simulink model "gm_rgbFilter_2024a"  (R2024a)
settings: Solver=FixedStepDiscrete  StartTime=0.0  StopTime=2  RelTol=1e-3
undefined symbols (not defined in the file or in its folder): blueMax, gray, greenMax, redMax
libraries: hdlsllib x13, visionhdlio x3, visionsources x1
Description:
  | Sobel Edge Detection Using the MATLAB(R) Function Block
  | This example shows how to use HDL Coder(TM) to check,
  | generate, and verify HDL code for a Sobel Edge Detection
  | block built using the MATLAB Function block.
settings Model: FPTRunName=Active  Creator=The MathWorks, Inc.  LastModifiedBy=dskiee
settings SolverCC: AlgebraicLoopSolver=TrustRegion
settings DataIOCC: LimitDataPoints=on  SaveFormat=Array  SignalLogging=off  ReturnWorkspaceOutputs=off
settings OptimizationCC: BlockReduction=off  ConditionallyExecuteInputs=off  DefaultParameterBehavior=Inlined  ExpressionDepthLimit=2147483647  InitFltsAndDblsToZero=on  EfficientMapNaN2IntZero=off  LifeSpan=inf
settings DebuggingCC: AlgebraicLoopMsg=error  SaveWithParameterizedLinksMsg=none  UnderspecifiedInitializationDetection=Classic  MergeDetectMultiDrivingBlocksExec=none  SignalResolutionControl=TryResolveAllWithWarning  InheritedTsInSrcMsg=none  MultiTaskDSMMsg=warning  MultiTaskCondExecSysMsg=none  SingleTaskRateTransMsg=error  IntegerOverflowMsg=none  ParameterPrecisionLossMsg=none  FcnCallInpInsideContextMsg=warning  UnconnectedInputMsg=warning  UnconnectedOutputMsg=warning  UnconnectedLineMsg=warning  AllowSymbolicDim=off  StateNameClashWarn=warning  StrictBusMsg=ErrorOnBusTreatedAsVector  SFUnexpectedBacktrackingDiag=warning  SFNoUnconditionalDefaultTransitionDiag=warning  SFExecutionAtInitializationDiag=none  IntegerSaturationMsg=none  ArithmeticOperatorsInVariantConditions=warning
settings HardwareCC: ProdBitPerPointer=32  ProdBitPerSizeT=32  ProdBitPerPtrDiffT=32  ProdLargestAtomicFloat=None  ProdIntDivRoundTo=Undefined  ProdEndianess=Unspecified  ProdWordSize=32  ProdHWDeviceType=ASIC/FPGA  TargetHWDeviceType=32-bit Generic  ProdEqTarget=off
settings ModelReferenceCC: EnableRefExpFcnMdlSchedulingChecks=on  PropagateSignalLabelsOutOfModel=off
settings SFSimCC: SimUseLocalCustomCode=off  CustomCodeUndefinedFunction=UseInterfaceOnly
settings RTWCC: RTWUseLocalCustomCode=off  GPUComputeCapability=3.5  DLArmComputeVersion=19.05
settings CodeAppCC: StateflowObjectComments=on
settings GRTTargetCC: TargetFcnLib=ansi_tfl_tmw.mat  TargetLangStandard=C89/C90 (ANSI)  CombineOutputUpdateFcns=off  GRTInterface=on
settings ConfigComp: CovMetricSettings=dw  CovSaveCumulativeToWorkspaceVar=on  CovSaveSingleToWorkspaceVar=on  CovExternalEMLEnable=off

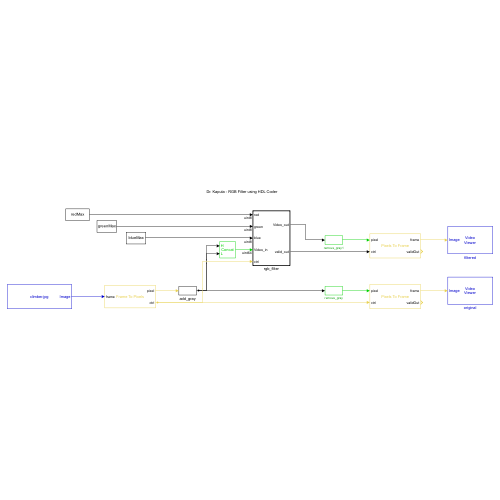
[thumbnail: Simulink's stored preview of the top-level diagram]
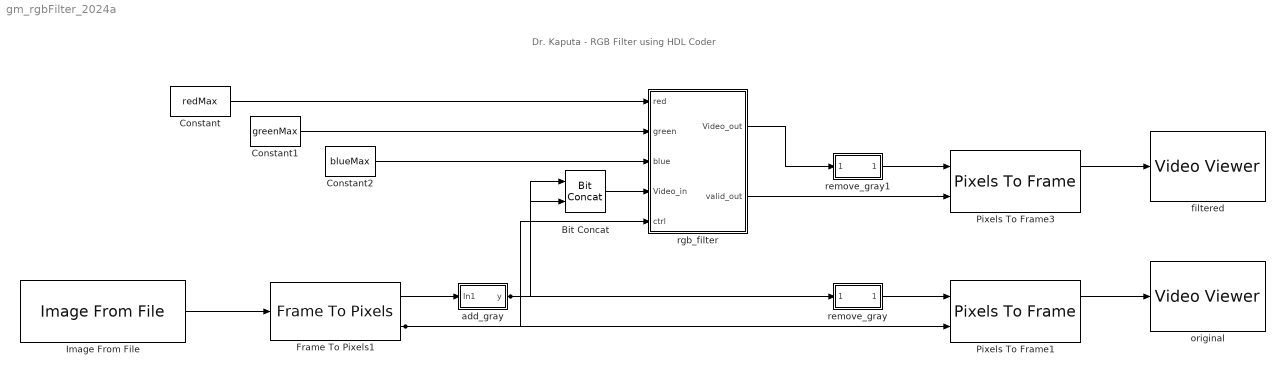
== system gm_rgbFilter_2024a ==
  note: Dr. Kaputa - RGB Filter using HDL Coder
  Bit Concat : hdlsllib/Logic and Bit Operations/Bit Concat  numInputs=2
  Constant : Constant  Value=redMax  OutDataTypeStr=uint8  SampleTime=-1
  Constant1 : Constant  Value=greenMax  OutDataTypeStr=uint8  SampleTime=-1
  Constant2 : Constant  Value=blueMax  OutDataTypeStr=uint8  SampleTime=-1
  Frame To Pixels1 : visionhdlio/Frame To Pixels  NumComponents=3  NumPixels=1  VideoFormat=Custom  ActivePixelsPerLine=R  ActiveVideoLines=C  TotalPixelsPerLine=R  TotalVideoLines=C  StartingActiveLine=1  FrontPorch=0  SampleTime=0  VideoFormatCache=Custom  ActivePixelsPerLineCache=R  ActiveVideoLinesCache=C  TotalPixelsPerLineCache=R  TotalVideoLinesCache=C  StartingActiveLineCache=1  FrontPorchCache=0
  Image From File : visionsources/Image From File  Tag=vipblks_nd  FileName=climber.jpg  Ts=1  imagePorts=One multidimensional signal  OutPortLabels=R|G|B  ImageDataType=Inherit from input image  sdImageDataType=uint(8)  Signed=on  WordLength=16  FractionLengthMode=User-defined  FractionLength=15
  Pixels To Frame1 : visionhdlio/Pixels To Frame  NumComponents=3  NumPixels=1  VideoFormat=Custom  ActivePixelsPerLine=R  ActiveVideoLines=C  TotalPixelsPerLine=R  TotalVideoLines=C  VideoFormatCache=Custom  ActivePixelsPerLineCache=R  ActiveVideoLinesCache=C  TotalPixelsPerLineCache=R  TotalVideoLinesCache=C
  Pixels To Frame3 : visionhdlio/Pixels To Frame  NumComponents=3  NumPixels=1  VideoFormat=Custom  ActivePixelsPerLine=R  ActiveVideoLines=C  TotalPixelsPerLine=R  TotalVideoLines=C  VideoFormatCache=Custom  ActivePixelsPerLineCache=R  ActiveVideoLinesCache=C  TotalPixelsPerLineCache=R  TotalVideoLinesCache=C
  add_gray : Subsystem
  filtered : VideoViewer  colormapValue=gray(256)  FigPos=[-1034.33333333333 813.333333333333 1280 622.666666666667]
  original : VideoViewer  FigPos=[-1388.33333333333 754 1280 622.666666666667]
  remove_gray : Subsystem
  remove_gray1 : Subsystem
  rgb_filter : Subsystem  TreatAsAtomicUnit=on
  wires:
  Constant2/1 -> rgb_filter/3(blue)
  Constant1/1 -> rgb_filter/2(green)
  Constant/1 -> rgb_filter/1(red)
  remove_gray1/1(RGBVector) -> Pixels To Frame3/1
  Bit Concat/1 -> rgb_filter/4(Video_in)
  rgb_filter/2(valid_out) -> Pixels To Frame3/2
  rgb_filter/1(Video_out) -> remove_gray1/1(RGB)
  Pixels To Frame3/1 -> filtered/1
  add_gray/1(y) -> remove_gray/1(RGB), Bit Concat/2, Bit Concat/1
  Frame To Pixels1/1 -> add_gray/1(In1)
  remove_gray/1(RGBVector) -> Pixels To Frame1/1
  Frame To Pixels1/2 -> Pixels To Frame1/2, rgb_filter/5(ctrl)
  Pixels To Frame1/1 -> original/1
  Image From File/1 -> Frame To Pixels1/1

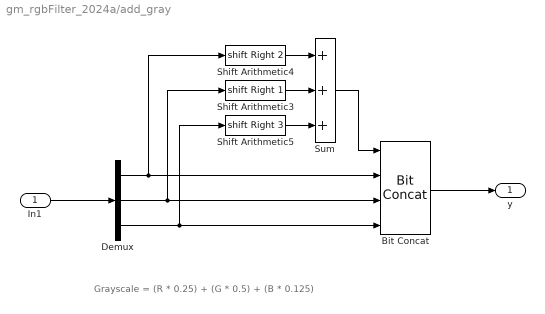
== system gm_rgbFilter_2024a/add_gray ==
  note: Grayscale = (R * 0.25) + (G * 0.5) + (B * 0.125)
  In1 : Inport
  Bit Concat : hdlsllib/Logic and Bit Operations/Bit Concat  numInputs=4
  Demux : Demux  Outputs=3
  Shift Arithmetic3 : ArithShift  BitShiftNumber=1  BitShiftDirection=Right
  Shift Arithmetic4 : ArithShift  BitShiftNumber=2  BitShiftDirection=Right
  Shift Arithmetic5 : ArithShift  BitShiftNumber=3  BitShiftDirection=Right
  Sum : Sum  Inputs=+++  OutDataTypeStr=uint8
  y : Outport
  wires:
  Shift Arithmetic5/1 -> Sum/3
  Shift Arithmetic3/1 -> Sum/2
  Shift Arithmetic4/1 -> Sum/1
  Sum/1 -> Bit Concat/1
  Demux/3 -> Bit Concat/4, Shift Arithmetic5/1
  Demux/1 -> Bit Concat/2, Shift Arithmetic4/1
  Demux/2 -> Bit Concat/3, Shift Arithmetic3/1
  In1/1 -> Demux/1
  Bit Concat/1 -> y/1

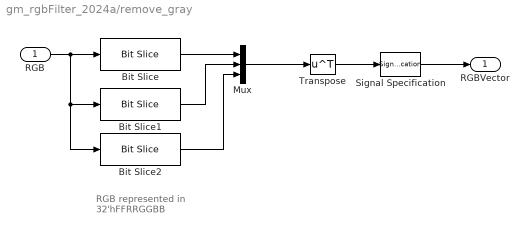
== system gm_rgbFilter_2024a/remove_gray ==
  note: RGB represented in
      | 32'hFFRRGGBB
  RGB : Inport
  Bit Slice : hdlsllib/Logic and Bit Operations/Bit Slice  lidx=23  ridx=16
  Bit Slice1 : hdlsllib/Logic and Bit Operations/Bit Slice  lidx=15  ridx=8
  Bit Slice2 : hdlsllib/Logic and Bit Operations/Bit Slice  lidx=7  ridx=0
  Mux : Mux  Inputs=3
  Signal Specification : SignalSpecification
  Transpose : Math  Operator=transpose  SignedPower=on
  RGBVector : Outport  VectorParamsAs1DForOutWhenUnconnected=off
  wires:
  Mux/1 -> Transpose/1
  Bit Slice/1 -> Mux/1
  Bit Slice2/1 -> Mux/3
  Bit Slice1/1 -> Mux/2
  RGB/1 -> Bit Slice2/1, Bit Slice1/1, Bit Slice/1
  Transpose/1 -> Signal Specification/1
  Signal Specification/1 -> RGBVector/1

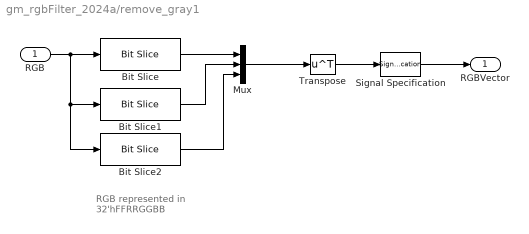
== system gm_rgbFilter_2024a/remove_gray1 ==
  note: RGB represented in
      | 32'hFFRRGGBB
  RGB : Inport
  Bit Slice : hdlsllib/Logic and Bit Operations/Bit Slice  lidx=23  ridx=16
  Bit Slice1 : hdlsllib/Logic and Bit Operations/Bit Slice  lidx=15  ridx=8
  Bit Slice2 : hdlsllib/Logic and Bit Operations/Bit Slice  lidx=7  ridx=0
  Mux : Mux  Inputs=3
  Signal Specification : SignalSpecification
  Transpose : Math  Operator=transpose  SignedPower=on
  RGBVector : Outport  VectorParamsAs1DForOutWhenUnconnected=off
  wires:
  Mux/1 -> Transpose/1
  Bit Slice/1 -> Mux/1
  Bit Slice2/1 -> Mux/3
  Bit Slice1/1 -> Mux/2
  RGB/1 -> Bit Slice2/1, Bit Slice1/1, Bit Slice/1
  Transpose/1 -> Signal Specification/1
  Signal Specification/1 -> RGBVector/1

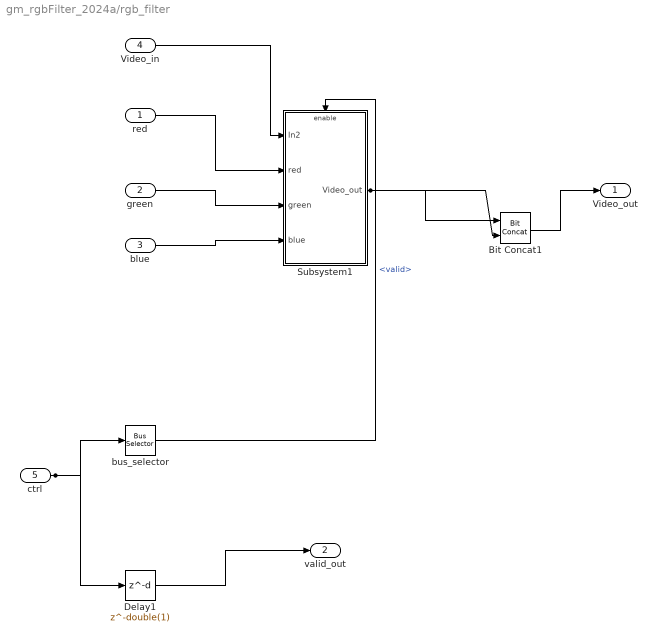
== system gm_rgbFilter_2024a/rgb_filter ==
  red : Inport  OutDataTypeStr=uint8  PortDimensions=1  SampleTime=2.77039007092199e-06
  green : Inport  Port=2  OutDataTypeStr=uint8  PortDimensions=1  SampleTime=2.77039007092199e-06
  blue : Inport  Port=3  OutDataTypeStr=uint8  PortDimensions=1  SampleTime=2.77039007092199e-06
  Video_in : Inport  Port=4  OutDataTypeStr=fixdt(0, 64, 0)  PortDimensions=1  SampleTime=2.77039007092199e-06
  ctrl : Inport  Port=5
  Bit Concat1 : hdlsllib/Logic and Bit Operations/Bit Concat  numInputs=2
  Delay1 : Delay  DelayLength=double(1)  SampleTime=2.77039007092199e-06
  Subsystem1 : Subsystem
  bus_selector : BusSelector  OutputSignals=valid
  Video_out : Outport  SampleTime=2.77039007092199e-06  VectorParamsAs1DForOutWhenUnconnected=off
  valid_out : Outport  Port=2  VectorParamsAs1DForOutWhenUnconnected=off
  wires:
  red/1 -> Subsystem1/2(red)
  green/1 -> Subsystem1/3(green)
  blue/1 -> Subsystem1/4(blue)
  Video_in/1 -> Subsystem1/1(In2)
  ctrl/1 -> bus_selector/1, Delay1/1
  Bit Concat1/1 -> Video_out/1
  bus_selector/1 -> Subsystem1/Enable  "<valid>"
  Delay1/1 -> valid_out/1
  Subsystem1/1(Video_out) -> Bit Concat1/2, Bit Concat1/1

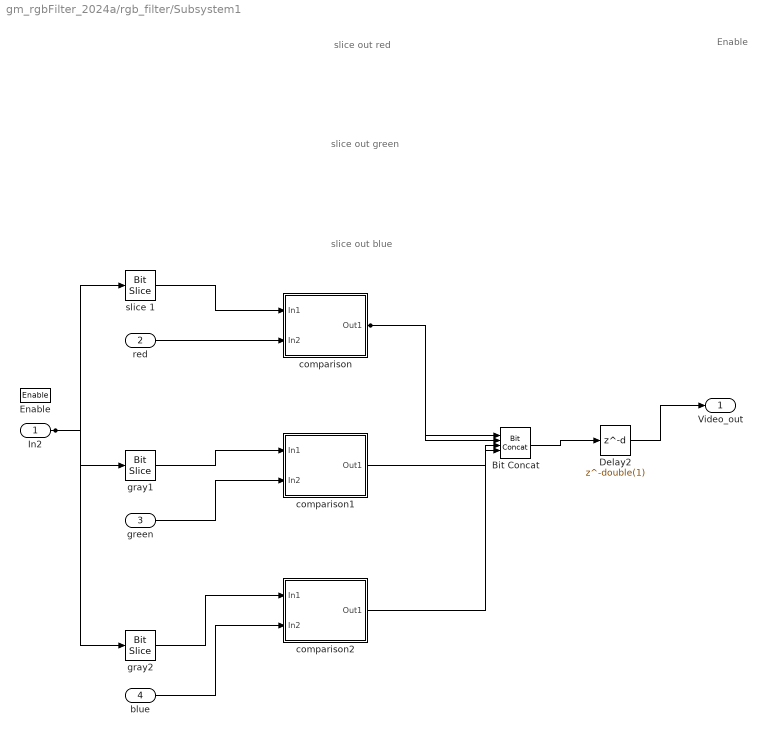
== system gm_rgbFilter_2024a/rgb_filter/Subsystem1 ==
  note: Enable
  note: slice out blue
  note: slice out green
  note: slice out red
  In2 : Inport  OutDataTypeStr=fixdt(0, 64, 0)  PortDimensions=1  SampleTime=2.77039007092199e-06
  red : Inport  Port=2  OutDataTypeStr=uint8  PortDimensions=1  SampleTime=2.77039007092199e-06
  green : Inport  Port=3  OutDataTypeStr=uint8  PortDimensions=1  SampleTime=2.77039007092199e-06
  blue : Inport  Port=4  OutDataTypeStr=uint8  PortDimensions=1  SampleTime=2.77039007092199e-06
  Enable : EnablePort  OutDataTypeStr=boolean
  Bit Concat : hdlsllib/Logic and Bit Operations/Bit Concat  numInputs=4
  Delay2 : Delay  DelayLength=double(1)  InitialCondition=0
  comparison : Subsystem
  comparison1 : Subsystem
  comparison2 : Subsystem
  gray1 : hdlsllib/Logic and Bit Operations/Bit Slice  lidx=double(15)  ridx=double(8)
  gray2 : hdlsllib/Logic and Bit Operations/Bit Slice  lidx=double(7)  ridx=double(0)
  slice 1 : hdlsllib/Logic and Bit Operations/Bit Slice  lidx=double(23)  ridx=double(16)
  Video_out : Outport  SampleTime=2.77039007092199e-06  InitialOutput=0
  wires:
  In2/1 -> slice 1/1, gray2/1, gray1/1
  red/1 -> comparison/2(In2)
  green/1 -> comparison1/2(In2)
  blue/1 -> comparison2/2(In2)
  Bit Concat/1 -> Delay2/1
  Delay2/1 -> Video_out/1
  comparison/1(Out1) -> Bit Concat/2, Bit Concat/1
  comparison1/1(Out1) -> Bit Concat/3
  comparison2/1(Out1) -> Bit Concat/4
  gray1/1 -> comparison1/1(In1)
  gray2/1 -> comparison2/1(In1)
  slice 1/1 -> comparison/1(In1)

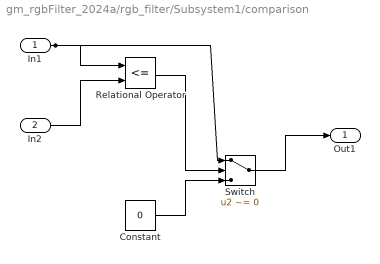
== system gm_rgbFilter_2024a/rgb_filter/Subsystem1/comparison ==
  In1 : Inport  OutDataTypeStr=uint8  PortDimensions=1  SampleTime=2.77039007092199e-06
  In2 : Inport  Port=2  OutDataTypeStr=uint8  PortDimensions=1  SampleTime=2.77039007092199e-06
  Constant : Constant  Value=0  OutDataTypeStr=uint8  SampleTime=2.77039007092199e-06
  Relational Operator : RelationalOperator  Operator=<=  OutDataTypeStr=boolean  SampleTime=2.77039007092199e-06  InputSameDT=off
  Switch : Switch  Criteria=u2 ~= 0  Threshold=double(0)  OutDataTypeStr=uint8  SampleTime=2.77039007092199e-06  SaturateOnIntegerOverflow=off  InputSameDT=off
  Out1 : Outport  SampleTime=2.77039007092199e-06  InitialOutput=0
  wires:
  In1/1 -> Switch/1, Relational Operator/1
  In2/1 -> Relational Operator/2
  Constant/1 -> Switch/3
  Relational Operator/1 -> Switch/2
  Switch/1 -> Out1/1

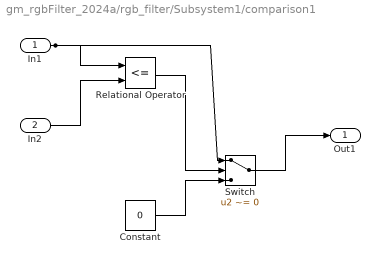
== system gm_rgbFilter_2024a/rgb_filter/Subsystem1/comparison1 ==
  In1 : Inport  OutDataTypeStr=uint8  PortDimensions=1  SampleTime=2.77039007092199e-06
  In2 : Inport  Port=2  OutDataTypeStr=uint8  PortDimensions=1  SampleTime=2.77039007092199e-06
  Constant : Constant  Value=0  OutDataTypeStr=uint8  SampleTime=2.77039007092199e-06
  Relational Operator : RelationalOperator  Operator=<=  OutDataTypeStr=boolean  SampleTime=2.77039007092199e-06  InputSameDT=off
  Switch : Switch  Criteria=u2 ~= 0  Threshold=double(0)  OutDataTypeStr=uint8  SampleTime=2.77039007092199e-06  SaturateOnIntegerOverflow=off  InputSameDT=off
  Out1 : Outport  SampleTime=2.77039007092199e-06  InitialOutput=0
  wires:
  In1/1 -> Switch/1, Relational Operator/1
  In2/1 -> Relational Operator/2
  Constant/1 -> Switch/3
  Relational Operator/1 -> Switch/2
  Switch/1 -> Out1/1

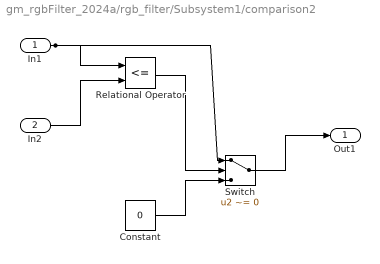
== system gm_rgbFilter_2024a/rgb_filter/Subsystem1/comparison2 ==
  In1 : Inport  OutDataTypeStr=uint8  PortDimensions=1  SampleTime=2.77039007092199e-06
  In2 : Inport  Port=2  OutDataTypeStr=uint8  PortDimensions=1  SampleTime=2.77039007092199e-06
  Constant : Constant  Value=0  OutDataTypeStr=uint8  SampleTime=2.77039007092199e-06
  Relational Operator : RelationalOperator  Operator=<=  OutDataTypeStr=boolean  SampleTime=2.77039007092199e-06  InputSameDT=off
  Switch : Switch  Criteria=u2 ~= 0  Threshold=double(0)  OutDataTypeStr=uint8  SampleTime=2.77039007092199e-06  SaturateOnIntegerOverflow=off  InputSameDT=off
  Out1 : Outport  SampleTime=2.77039007092199e-06  InitialOutput=0
  wires:
  In1/1 -> Switch/1, Relational Operator/1
  In2/1 -> Relational Operator/2
  Constant/1 -> Switch/3
  Relational Operator/1 -> Switch/2
  Switch/1 -> Out1/1
